simulink model "VFA_pomucka"  (R2021b)
settings: Solver=ode4  StartTime=0.0  StopTime=10.0  FixedStep=Ts  RelTol=1e-3  EnableMultiTasking=on
values from neighbouring files (symbols this model uses):
  A = 5    [init_VFA.m]
  f = 400    [init_VFA.m]
  numT = 20    [init_VFA.m]
  offset = 6    [init_VFA.m]
  T = 1/f    (= 0.0025)    [init_VFA.m]
  Ts = 125e-6    (= 0.000125)    [init_VFA.m]
libraries: simulink x3
settings Model: Creator=Vesely  LastModifiedBy=239026
settings SolverCC: AlgebraicLoopSolver=TrustRegion
settings DataIOCC: LimitDataPoints=on  SaveFormat=Array  SignalLoggingSaveFormat=ModelDataLogs  ReturnWorkspaceOutputs=off
settings OptimizationCC: ExpressionDepthLimit=2147483647  LifeSpan=inf
settings DebuggingCC: UnderspecifiedInitializationDetection=Classic  MergeDetectMultiDrivingBlocksExec=none  SolverPrmCheckMsg=warning  FcnCallInpInsideContextMsg=warning  AllowSymbolicDim=off  StateNameClashWarn=warning  SFUnexpectedBacktrackingDiag=warning  SFNoUnconditionalDefaultTransitionDiag=warning  SFExecutionAtInitializationDiag=none  SFMachineParentedDataDiag=warning  ArithmeticOperatorsInVariantConditions=warning
settings HardwareCC: ProdBitPerPointer=32  ProdBitPerSizeT=32  ProdBitPerPtrDiffT=32  ProdLargestAtomicFloat=None  ProdIntDivRoundTo=Undefined  ProdEndianess=Unspecified  ProdWordSize=32  ProdHWDeviceType=32-bit Generic
settings ModelReferenceCC: PropagateSignalLabelsOutOfModel=off
settings SFSimCC: SimUseLocalCustomCode=off  CustomCodeUndefinedFunction=UseInterfaceOnly
settings RTWCC: RTWUseLocalCustomCode=off
settings CodeAppCC: StateflowObjectComments=on
settings GRTTargetCC: TargetLangStandard=C89/C90 (ANSI)  CombineOutputUpdateFcns=off  GRTInterface=on
settings ConfigComp: CovMetricSettings=dw  CovSaveCumulativeToWorkspaceVar=on  CovSaveSingleToWorkspaceVar=on  CovExternalEMLEnable=off

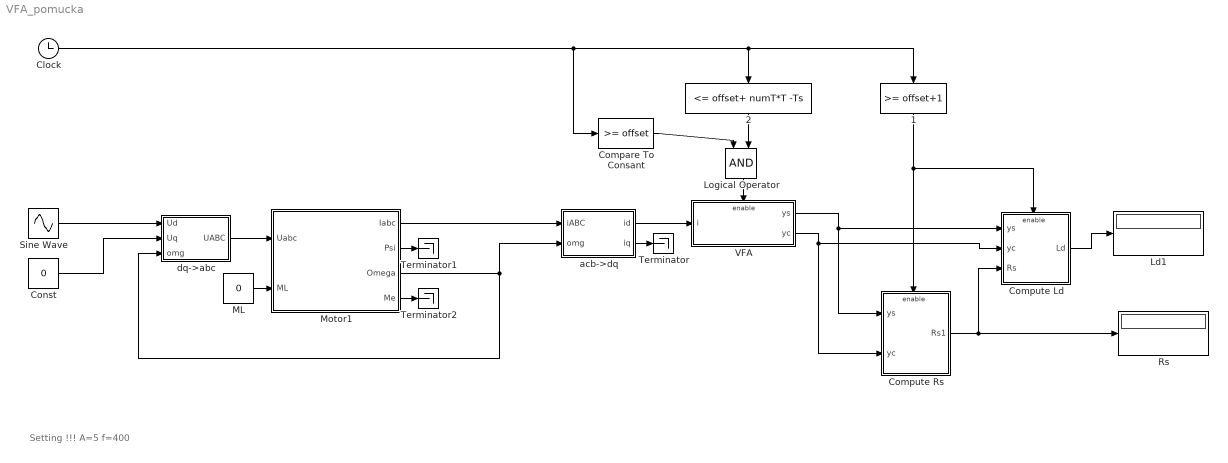
== system VFA_pomucka ==
  note: Setting !!!
      | A=5
      | f=400
  1 : simulink/Logic and Bit Operations/Compare To Constant  relop=>=  const=offset+1  OutDataTypeStr=boolean  ZeroCross=off
  2 : simulink/Logic and Bit Operations/Compare To Constant  relop=<=  const=offset+ numT*T -Ts  OutDataTypeStr=boolean  ZeroCross=off
  Clock : Clock
  Compare To Consant : simulink/Logic and Bit Operations/Compare To Constant  relop=>=  const=offset  OutDataTypeStr=boolean  ZeroCross=off
  Compute Ld : Subsystem  TreatAsAtomicUnit=on
  Compute Rs : Subsystem  TreatAsAtomicUnit=on
  Const : Constant  Value=0
  Ld1 : Display
  Logical Operator : Logic  AllPortsSameDT=off  OutDataTypeStr=boolean
  ML : Constant  Value=0
  Motor1 : Subsystem  mask{Rs=0.14, Ld=1.29e-3, Lq=1.29e-3, p=3, J=0.0104, PSIb=0.378}
      mask prompts: Rs "Cinny odpor statorove faze"; Ld "Indukcnost v podelne ose"; Lq "Indukcnost v pricne ose"; p "Pocet polovych dvojic"; J "Celkovy moment setrvacnosti"; PSIb "Magneticky tok magnetu"
      mask Display:
      | plot(0,0,100,100,[40,70,72,73,73,73,72,70,40,37,36,36,36,37,40,43,44,44,44,43,40],[30,30,32,40,50,60,67,70,70,67,60,50,40,33,30,33,40,50,60,67,70],[40,20,21,20,40,41,40],[51,51,50,48,48,50,51],[20,19,20],[48,50,51],[52,52,46,46],[30,27,27,30],[64,64,58,58],[30,27,27,30],[70,47],[60,60],[70,47],[50,50],[70,47],[40,40],[69,46],[65,65],[70,47],[55,55],[70,47],[45,45],[69,46],[35,35],[20,20,21,23,24,24,23,22,20],[44,40,42,45,50,53,56,59,60],[23,20],[40,40])
      | color('black')
      | text(25,90,'Synch Motor')
      | color('black')
      | port_label('input',1,'u_{A,B,C}', 'texmode', 'on');
      | port_label('input',2,'ML', 'texmode', 'on');
      | port_label('output',1,'i_{A,B,C}', 'texmode', 'on');
      | port_label('output',2,'\Psi', 'texmode', 'on');
      | port_label('output',3,'\omega', 'texmode', 'on');
      | port_label('output',4,'M_e', 'texmode', 'on');
  Rs : Display
  Sine Wave : Sin  Amplitude=A  Frequency=2*pi*f  SampleTime=0
  Terminator : Terminator
  Terminator1 : Terminator
  Terminator2 : Terminator
  VFA : Subsystem  TreatAsAtomicUnit=on
  acb->dq : Subsystem  TreatAsAtomicUnit=on
  dq->abc : Subsystem
  wires:
  Sine Wave/1 -> dq->abc/1(Ud)
  Motor1/3(Omega) -> dq->abc/3(omg), acb->dq/2(omg)
  ML/1 -> Motor1/2(ML)
  dq->abc/1(UABC) -> Motor1/1(Uabc)
  Clock/1 -> Compare To Consant/1, 2/1, 1/1
  Compare To Consant/1 -> Logical Operator/1
  2/1 -> Logical Operator/2
  acb->dq/1(id) -> VFA/1(i)
  Logical Operator/1 -> VFA/Enable
  1/1 -> Compute Ld/Enable, Compute Rs/Enable
  VFA/1(ys) -> Compute Ld/1(ys), Compute Rs/1(ys)
  VFA/2(yc) -> Compute Ld/2(yc), Compute Rs/2(yc)
  Compute Ld/1(Ld) -> Ld1/1
  Compute Rs/1(Rs1) -> Rs/1, Compute Ld/3(Rs)
  Motor1/1(Iabc) -> acb->dq/1(iABC)
  Const/1 -> dq->abc/2(Uq)
  Motor1/2(Psi) -> Terminator1/1
  Motor1/4(Me) -> Terminator2/1
  acb->dq/2(iq) -> Terminator/1

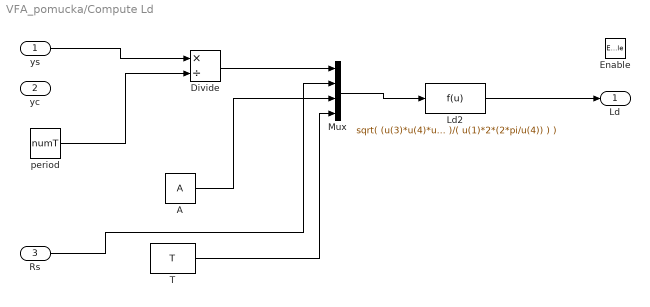
== system VFA_pomucka/Compute Ld ==
  ys : Inport
  yc : Inport  Port=2
  Rs : Inport  Port=3
  Enable : EnablePort
  A : Constant  Value=A
  Divide : Product  Inputs=*/
  Ld2 : Fcn  Expr=sqrt( (u(3)*u(4)*u(2) - u(1)*2*u(2)^2 )/( u(1)*2*(2*pi/u(4)) ) )
  Mux : Mux
  T : Constant  Value=T
  period : Constant  Value=numT
  Ld : Outport
  wires:
  Ld2/1 -> Ld/1
  Mux/1 -> Ld2/1
  period/1 -> Divide/2
  ys/1 -> Divide/1
  T/1 -> Mux/4
  A/1 -> Mux/3
  Divide/1 -> Mux/1
  Rs/1 -> Mux/2

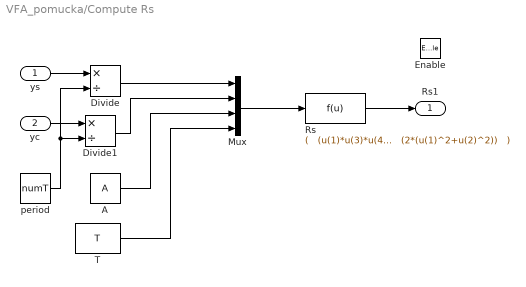
== system VFA_pomucka/Compute Rs ==
  ys : Inport
  yc : Inport  Port=2
  Enable : EnablePort  PropagateVarSize=During execution
  A : Constant  Value=A
  Divide : Product  Inputs=*/
  Divide1 : Product  Inputs=*/
  Mux : Mux
  Rs : Fcn  Expr="(   (u(1)*u(3)*u(4))   /   (2*(u(1)^2+u(2)^2))   )"
  T : Constant  Value=T
  period : Constant  Value=numT
  Rs1 : Outport
  wires:
  Rs/1 -> Rs1/1
  period/1 -> Divide/2, Divide1/2
  Mux/1 -> Rs/1
  yc/1 -> Divide1/1
  ys/1 -> Divide/1
  Divide/1 -> Mux/1
  Divide1/1 -> Mux/2
  T/1 -> Mux/4
  A/1 -> Mux/3

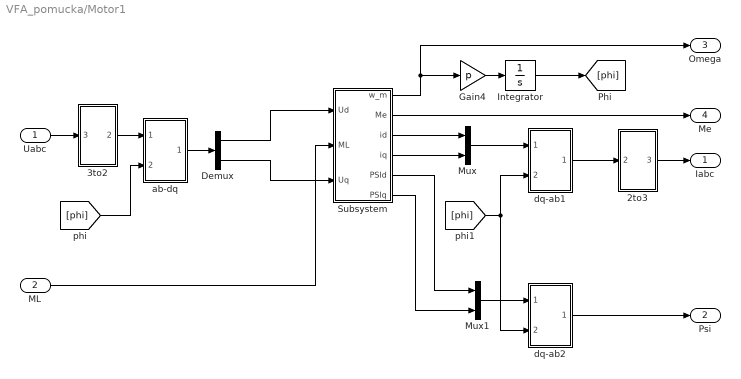
== system VFA_pomucka/Motor1 ==
  Uabc : Inport
  ML : Inport  Port=2
  2to3 : Subsystem
      mask help: 2 ph to 3 ph transformation
      mask Display: disp('2 > 3')
  3to2 : Subsystem
      mask help: 3 ph to 2 ph transformation
      mask Display: disp('3 > 2')
  Demux : Demux  Outputs=2
  Gain4 : Gain  Gain=p
  Integrator : Integrator
  Mux : Mux  Inputs=2
  Mux1 : Mux  Inputs=2
  Subsystem : Subsystem
  ab-dq : Subsystem
  dq-ab1 : Subsystem
  dq-ab2 : Subsystem
  Iabc : Outport
  Psi : Outport  Port=2
  Omega : Outport  Port=3
  Me : Outport  Port=4
  wires:
  Gain4/1 -> Integrator/1
  dq-ab1/1(x_ab) -> 2to3/1(2)
  Mux/1 -> dq-ab1/1(x_dq)
  [phi] -> dq-ab2/2(phi), dq-ab1/2(phi)
  [phi] -> ab-dq/2(phi)
  Integrator/1 -> [phi]
  ab-dq/1(x_dq) -> Demux/1
  3to2/1(2) -> ab-dq/1(x_ab)
  Demux/1 -> Subsystem/1(Ud)
  Demux/2 -> Subsystem/3(Uq)
  ML/1 -> Subsystem/2(ML)
  Subsystem/3(id) -> Mux/1
  Subsystem/4(iq) -> Mux/2
  Uabc/1 -> 3to2/1(3)
  Subsystem/5(PSId) -> Mux1/1
  Mux1/1 -> dq-ab2/1(x_dq)
  Subsystem/6(PSIq) -> Mux1/2
  2to3/1(3) -> Iabc/1
  dq-ab2/1(x_ab) -> Psi/1
  Subsystem/1(w_m) -> Gain4/1, Omega/1
  Subsystem/2(Me) -> Me/1

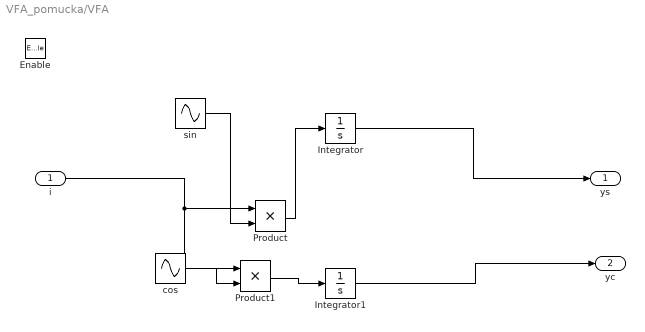
== system VFA_pomucka/VFA ==
  i : Inport  SampleTime=125e-6
  Enable : EnablePort  StatesWhenEnabling=reset
  Integrator : Integrator
  Integrator1 : Integrator
  Product : Product
  Product1 : Product
  cos : Sin  Frequency=2*pi*f  Phase=pi/2
  sin : Sin  Frequency=2*pi*f  SampleTime=0
  ys : Outport
  yc : Outport  Port=2
  wires:
  Integrator/1 -> ys/1
  Integrator1/1 -> yc/1
  sin/1 -> Product/2
  i/1 -> Product/1, Product1/1
  Product/1 -> Integrator/1
  cos/1 -> Product1/2
  Product1/1 -> Integrator1/1

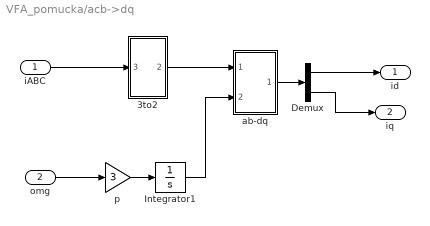
== system VFA_pomucka/acb->dq ==
  iABC : Inport
  omg : Inport  Port=2
  3to2 : Subsystem
      mask help: 3 ph to 2 ph transformation
      mask Display: disp('3 > 2')
  Demux : Demux  Outputs=2
  Integrator1 : Integrator
  ab-dq : Subsystem
  p : Gain  Gain=3
  id : Outport
  iq : Outport  Port=2
  wires:
  Demux/2 -> iq/1
  Integrator1/1 -> ab-dq/2(phi)
  p/1 -> Integrator1/1
  omg/1 -> p/1
  Demux/1 -> id/1
  ab-dq/1(x_dq) -> Demux/1
  3to2/1(2) -> ab-dq/1(x_ab)
  iABC/1 -> 3to2/1(3)

== system VFA_pomucka/dq->abc ==
  Ud : Inport
  Uq : Inport  Port=2
  omg : Inport  Port=3
  2to3 : Subsystem
      mask help: 2 ph to 3 ph transformation
      mask Display: disp('2 > 3')
  Integrator1 : Integrator
  Mux : Mux  Inputs=2
  dq-ab1 : Subsystem
  p : Gain  Gain=3
  UABC : Outport
  wires:
  Uq/1 -> Mux/2
  Ud/1 -> Mux/1
  dq-ab1/1(x_ab) -> 2to3/1(2)
  Integrator1/1 -> dq-ab1/2(phi)
  p/1 -> Integrator1/1
  omg/1 -> p/1
  2to3/1(3) -> UABC/1
  Mux/1 -> dq-ab1/1(x_dq)

== system VFA_pomucka/Motor1/2to3 ==
  2 : Inport
  Matrix Gain : Gain  Gain=[1 0; -1/2 sqrt(3)/2; -1/2 -sqrt(3)/2]  Multiplication=Matrix(K*u)  SaturateOnIntegerOverflow=on  OutDataTypeStr=Inherit: Same as input  ParamDataTypeStr=Inherit: Same as input
  3 : Outport
  wires:
  Matrix Gain/1 -> 3/1
  2/1 -> Matrix Gain/1

== system VFA_pomucka/Motor1/3to2 ==
  3 : Inport
  Matrix Gain : Gain  Gain=[2/3 -1/3 -1/3 ; 0 1/sqrt(3) -1/sqrt(3)]  Multiplication=Matrix(K*u)  SaturateOnIntegerOverflow=on  OutDataTypeStr=Inherit: Same as input  ParamDataTypeStr=Inherit: Same as input
  2 : Outport
  wires:
  Matrix Gain/1 -> 2/1
  3/1 -> Matrix Gain/1

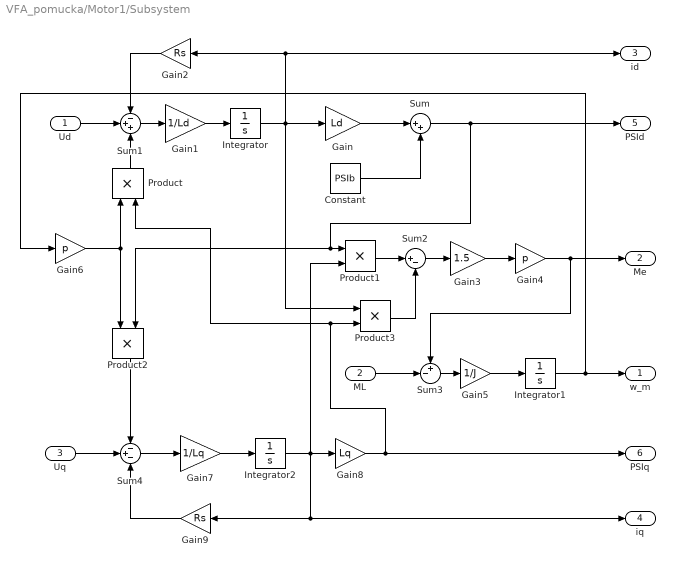
== system VFA_pomucka/Motor1/Subsystem ==
  Ud : Inport
  ML : Inport  Port=2
  Uq : Inport  Port=3
  Constant : Constant  Value=PSIb
  Gain : Gain  Gain=Ld
  Gain1 : Gain  Gain=1/Ld
  Gain2 : Gain  Gain=Rs
  Gain3 : Gain  Gain=1.5
  Gain4 : Gain  Gain=p
  Gain5 : Gain  Gain=1/J
  Gain6 : Gain  Gain=p
  Gain7 : Gain  Gain=1/Lq
  Gain8 : Gain  Gain=Lq
  Gain9 : Gain  Gain=Rs
  Integrator : Integrator
  Integrator1 : Integrator
  Integrator2 : Integrator
  Product{,1..3} (4 alike) : Product  RndMeth=Zero
  Sum : Sum  Inputs=|++
  Sum1 : Sum  Inputs=-++
  Sum2 : Sum  Inputs=|+-
  Sum3 : Sum  Inputs=+-|
  Sum4 : Sum  Inputs=-+-
  w_m : Outport
  Me : Outport  Port=2
  id : Outport  Port=3
  iq : Outport  Port=4
  PSId : Outport  Port=5
  PSIq : Outport  Port=6
  wires:
  Gain9/1 -> Sum4/3
  Gain8/1 -> Product/2, Product3/2, PSIq/1
  Integrator2/1 -> Product1/2, Gain9/1, iq/1, Gain8/1
  Gain7/1 -> Integrator2/1
  Sum4/1 -> Gain7/1
  Uq/1 -> Sum4/2
  Product2/1 -> Sum4/1
  Product3/1 -> Sum2/2
  Gain6/1 -> Product2/1, Product/1
  Integrator1/1 -> Gain6/1, w_m/1
  Gain5/1 -> Integrator1/1
  Sum3/1 -> Gain5/1
  ML/1 -> Sum3/2
  Gain4/1 -> Sum3/1, Me/1
  Gain3/1 -> Gain4/1
  Sum2/1 -> Gain3/1
  Product1/1 -> Sum2/1
  Sum/1 -> Product2/2, Product1/1, PSId/1
  Product/1 -> Sum1/3
  Ud/1 -> Sum1/2
  Gain2/1 -> Sum1/1
  Sum1/1 -> Gain1/1
  Gain1/1 -> Integrator/1
  Constant/1 -> Sum/2
  Gain/1 -> Sum/1
  Integrator/1 -> id/1, Gain2/1, Product3/1, Gain/1

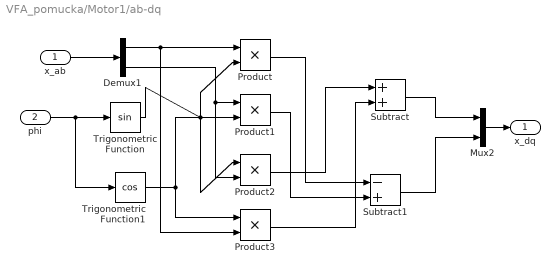
== system VFA_pomucka/Motor1/ab-dq ==
  x_ab : Inport
  phi : Inport  Port=2
  Demux1 : Demux  Outputs=2
  Mux2 : Mux  Inputs=2
  Product{,1..3} (4 alike) : Product  RndMeth=Zero
  Subtract : Sum
  Subtract1 : Sum  Inputs=-+
  Trigonometric Function : Trigonometry
  Trigonometric Function1 : Trigonometry  Operator=cos
  x_dq : Outport
  wires:
  Product1/1 -> Subtract1/2
  Product/1 -> Subtract1/1
  Product3/1 -> Subtract/2
  Product2/1 -> Subtract/1
  Trigonometric Function1/1 -> Product1/2, Product3/1
  Trigonometric Function/1 -> Product/2, Product2/1
  Demux1/2 -> Product2/2, Product1/1
  Demux1/1 -> Product3/2, Product/1
  phi/1 -> Trigonometric Function1/1, Trigonometric Function/1
  Subtract/1 -> Mux2/1
  Subtract1/1 -> Mux2/2
  x_ab/1 -> Demux1/1
  Mux2/1 -> x_dq/1

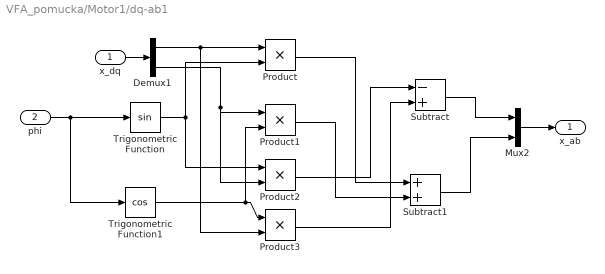
== system VFA_pomucka/Motor1/dq-ab1 ==
  x_dq : Inport
  phi : Inport  Port=2
  Demux1 : Demux  Outputs=2
  Mux2 : Mux  Inputs=2
  Product{,1..3} (4 alike) : Product  RndMeth=Zero
  Subtract : Sum  Inputs=-+
  Subtract1 : Sum
  Trigonometric Function : Trigonometry
  Trigonometric Function1 : Trigonometry  Operator=cos
  x_ab : Outport
  wires:
  Subtract1/1 -> Mux2/2
  Product3/1 -> Subtract/2
  Product2/1 -> Subtract/1
  Product1/1 -> Subtract1/2
  Product/1 -> Subtract1/1
  Trigonometric Function1/1 -> Product1/2, Product3/1
  Trigonometric Function/1 -> Product/2, Product2/1
  Demux1/2 -> Product2/2, Product1/1
  Demux1/1 -> Product3/2, Product/1
  phi/1 -> Trigonometric Function1/1, Trigonometric Function/1
  Subtract/1 -> Mux2/1
  x_dq/1 -> Demux1/1
  Mux2/1 -> x_ab/1

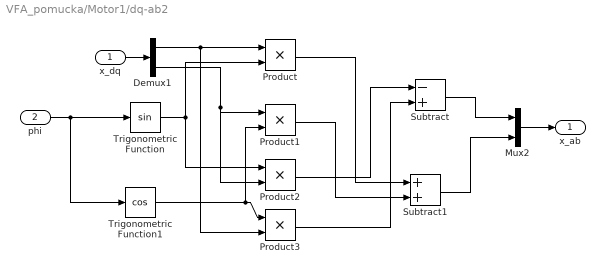
== system VFA_pomucka/Motor1/dq-ab2 ==
  x_dq : Inport
  phi : Inport  Port=2
  Demux1 : Demux  Outputs=2
  Mux2 : Mux  Inputs=2
  Product{,1..3} (4 alike) : Product  RndMeth=Zero
  Subtract : Sum  Inputs=-+
  Subtract1 : Sum
  Trigonometric Function : Trigonometry
  Trigonometric Function1 : Trigonometry  Operator=cos
  x_ab : Outport
  wires:
  Subtract1/1 -> Mux2/2
  Product3/1 -> Subtract/2
  Product2/1 -> Subtract/1
  Product1/1 -> Subtract1/2
  Product/1 -> Subtract1/1
  Trigonometric Function1/1 -> Product1/2, Product3/1
  Trigonometric Function/1 -> Product/2, Product2/1
  Demux1/2 -> Product2/2, Product1/1
  Demux1/1 -> Product3/2, Product/1
  phi/1 -> Trigonometric Function1/1, Trigonometric Function/1
  Subtract/1 -> Mux2/1
  x_dq/1 -> Demux1/1
  Mux2/1 -> x_ab/1

== system VFA_pomucka/acb->dq/3to2 ==
  3 : Inport
  Matrix Gain : Gain  Gain=[2/3 -1/3 -1/3 ; 0 1/sqrt(3) -1/sqrt(3)]  Multiplication=Matrix(K*u)  SaturateOnIntegerOverflow=on  OutDataTypeStr=Inherit: Same as input  ParamDataTypeStr=Inherit: Same as input
  2 : Outport
  wires:
  3/1 -> Matrix Gain/1
  Matrix Gain/1 -> 2/1

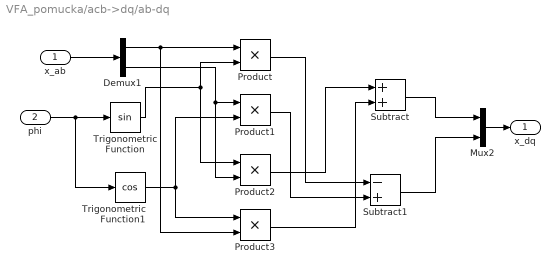
== system VFA_pomucka/acb->dq/ab-dq ==
  x_ab : Inport
  phi : Inport  Port=2
  Demux1 : Demux  Outputs=2
  Mux2 : Mux  Inputs=2
  Product{,1..3} (4 alike) : Product  RndMeth=Zero
  Subtract : Sum
  Subtract1 : Sum  Inputs=-+
  Trigonometric Function : Trigonometry
  Trigonometric Function1 : Trigonometry  Operator=cos
  x_dq : Outport
  wires:
  Product1/1 -> Subtract1/2
  Product/1 -> Subtract1/1
  Product3/1 -> Subtract/2
  Product2/1 -> Subtract/1
  Trigonometric Function1/1 -> Product1/2, Product3/1
  Trigonometric Function/1 -> Product/2, Product2/1
  Demux1/2 -> Product2/2, Product1/1
  Demux1/1 -> Product3/2, Product/1
  phi/1 -> Trigonometric Function1/1, Trigonometric Function/1
  Subtract/1 -> Mux2/1
  Subtract1/1 -> Mux2/2
  x_ab/1 -> Demux1/1
  Mux2/1 -> x_dq/1

== system VFA_pomucka/dq->abc/2to3 ==
  2 : Inport
  Matrix Gain : Gain  Gain=[1 0; -1/2 sqrt(3)/2; -1/2 -sqrt(3)/2]  Multiplication=Matrix(K*u)  SaturateOnIntegerOverflow=on  OutDataTypeStr=Inherit: Same as input  ParamDataTypeStr=Inherit: Same as input
  3 : Outport
  wires:
  2/1 -> Matrix Gain/1
  Matrix Gain/1 -> 3/1

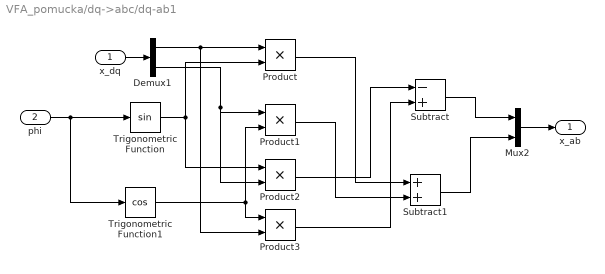
== system VFA_pomucka/dq->abc/dq-ab1 ==
  x_dq : Inport
  phi : Inport  Port=2
  Demux1 : Demux  Outputs=2
  Mux2 : Mux  Inputs=2
  Product{,1..3} (4 alike) : Product  RndMeth=Zero
  Subtract : Sum  Inputs=-+
  Subtract1 : Sum
  Trigonometric Function : Trigonometry
  Trigonometric Function1 : Trigonometry  Operator=cos
  x_ab : Outport
  wires:
  Subtract1/1 -> Mux2/2
  Product3/1 -> Subtract/2
  Product2/1 -> Subtract/1
  Product1/1 -> Subtract1/2
  Product/1 -> Subtract1/1
  Trigonometric Function1/1 -> Product3/1, Product1/2
  Trigonometric Function/1 -> Product/2, Product2/1
  Demux1/2 -> Product2/2, Product1/1
  Demux1/1 -> Product3/2, Product/1
  phi/1 -> Trigonometric Function1/1, Trigonometric Function/1
  Subtract/1 -> Mux2/1
  x_dq/1 -> Demux1/1
  Mux2/1 -> x_ab/1
